simulink model "EMK_Controller"  (R2021a)
settings: Solver=VariableStepAuto  StartTime=0.0  StopTime=10.0  RelTol=1e-3
settings Model: Creator=sahil  LastModifiedBy=sahil

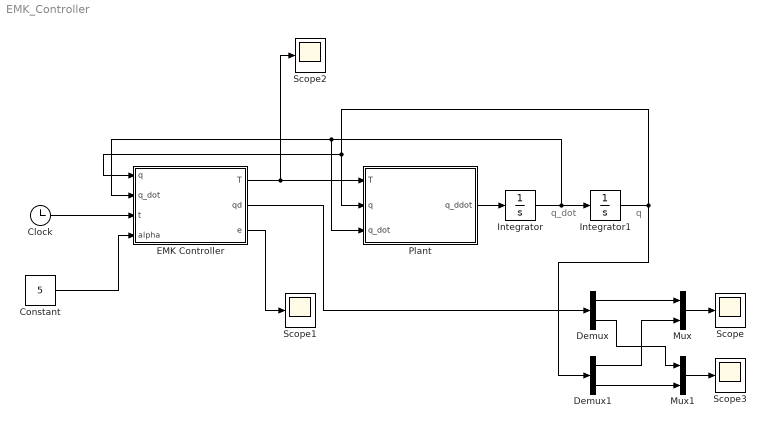
== system EMK_Controller ==
  note: q
  note: q_dot
  Clock : Clock
  Constant : Constant  Value=5
  Demux : Demux  Outputs=2
  Demux1 : Demux  Outputs=2
  EMK Controller : MATLAB Function  TreatAsAtomicUnit=on
  Integrator : Integrator  InitialCondition=[0; 0]
  Integrator1 : Integrator  InitialCondition=[0; 0]
  Mux : Mux  Inputs=2
  Mux1 : Mux  Inputs=2
  Plant : MATLAB Function  TreatAsAtomicUnit=on
  Scope{,1..3} (4 alike) : Scope
  wires:
  EMK Controller/2(qd) -> Demux/1
  Mux1/1 -> Scope3/1
  Demux/1 -> Mux/1
  Integrator/1 -> Plant/3(q_dot), EMK Controller/2(q_dot), Integrator1/1
  Demux/2 -> Mux1/1
  Integrator1/1 -> Demux1/1, Plant/2(q), EMK Controller/1(q)
  Clock/1 -> EMK Controller/3(t)
  Mux/1 -> Scope/1
  EMK Controller/1(T) -> Scope2/1, Plant/1(T)
  Demux1/2 -> Mux1/2
  EMK Controller/3(e) -> Scope1/1
  Plant/1(q_ddot) -> Integrator/1
  Demux1/1 -> Mux/2
  Constant/1 -> EMK Controller/4(alpha)

== matlab function EMK_Controller/EMK Controller ==
  data: q input; q_dot input; t input; T output; qd output; e output; alpha input
function [T, qd, e] = fcn(q, q_dot, t, alpha)
p1 = 3.473;
p2 = 0.196;
p3 = 0.242;
fd1 = 5.3;
fd2 = 1.1;
M = [(p1 + 2*p3*cos(q(2))) (p2 + p3*cos(q(2))); (p2 + p3*cos(q(2))) p2];
Vm = [(-p3*sin(q(2))*q_dot(2)) (-p3*sin(q(2))*(q_dot(1)+q_dot(2))); (p3*sin(q(2))*q_dot(1)) 0];
Fd = [fd1 0; 0 fd2];

%Control Gains
K = 20*eye(2);

%Desired trajectories
qd = [cos(t); cos(2*t)];
qd_dot = [-sin(t); -2*sin(2*t)];
qd_ddot = [-cos(t); -4*cos(2*t)];

%Errors
e = qd - q;
e_dot = qd_dot - q_dot;
r = e_dot + (alpha*e);

%EMK Controller
T = (M*qd_ddot) + (Vm*q_dot) + (Fd*q_dot) + (alpha*M*e_dot) + (Vm*r) + e + (K*r);

== matlab function EMK_Controller/Plant ==
  data: T input; q_ddot output; q input; q_dot input
function q_ddot = fcn(T, q, q_dot)
%Defining given parameters
p1 = 3.473;
p2 = 0.196;
p3 = 0.242;
fd1 = 5.3;
fd2 = 1.1;

%Defining Robot Dynamic Model
M = [(p1 + 2*p3*cos(q(2))) (p2 + p3*cos(q(2))); (p2 + p3*cos(q(2))) p2];
Vm = [(-p3*sin(q(2))*q_dot(2)) (-p3*sin(q(2))*(q_dot(1)+q_dot(2))); (p3*sin(q(2))*q_dot(1)) 0];
Fd = [fd1 0; 0 fd2];

%Robot Dynamics
q_ddot = inv(M)*(T - (Vm*q_dot) - (Fd*q_dot));
